simulink model "three_phase_npc_inverter"  (R2021a)
settings: Solver=ode4  StartTime=0.0  StopTime=0.1  FixedStep=1e-6  RelTol=1e-3
libraries: spsIGBTDiodeLib x12, spsDiodeLib x6, simulink x6, spsGroundLib x3, spsDCVoltageSourceLib x2, spsNeutralLib x1, spsThreePhaseSeriesRLCBranchLib x1, spsThreePhaseVIMeasurementLib x1, spspowerguiLib x1
settings Model: Creator=PRANAY KAMAL  LastModifiedBy=PRANAY KAMAL
settings DataIOCC: ReturnWorkspaceOutputs=off

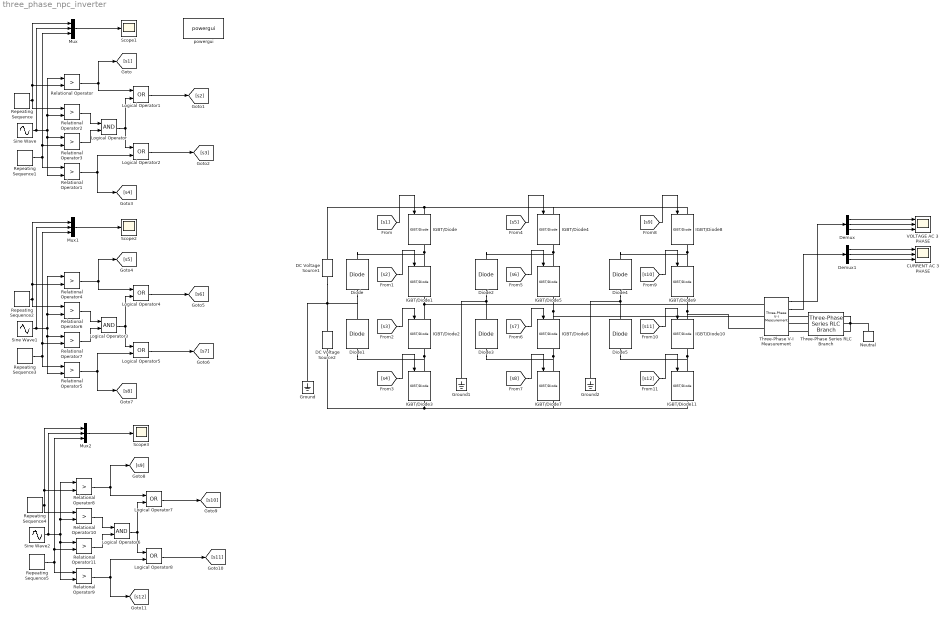
== system three_phase_npc_inverter ==
  CURRENT AC 3 PHASE : Scope  NumInputPorts=3
  DC Voltage Source1 : spsDCVoltageSourceLib/DC Voltage Source  Amplitude=200  Measurements=None
  DC Voltage Source2 : spsDCVoltageSourceLib/DC Voltage Source  Amplitude=200  Measurements=None
  Demux : Demux  Outputs=3
  Demux1 : Demux  Outputs=3
  Diode{,1..5} (6 alike) : spsDiodeLib/Diode  Ron=0.001  Lon=0  Vf=0.8  IC=0  UseSnubber=0  Rs=500  Cs=250e-9  Measurements=off
  Ground : spsGroundLib/Ground  LConnTagsString=a
  Ground1 : spsGroundLib/Ground  LConnTagsString=a
  Ground2 : spsGroundLib/Ground  LConnTagsString=a
  IGBT/Diode{,1..11} (12 alike) : spsIGBTDiodeLib/IGBT//Diode  Ron=1e-3  Rs=1e5  Cs=inf  Measurements=on
  Logical Operator : Logic  AllPortsSameDT=off  OutDataTypeStr=boolean
  Logical Operator{1..2,4..5,7..8} (6 alike) : Logic  Operator=OR  AllPortsSameDT=off  OutDataTypeStr=boolean
  Logical Operator3 : Logic  AllPortsSameDT=off  OutDataTypeStr=boolean
  Logical Operator6 : Logic  AllPortsSameDT=off  OutDataTypeStr=boolean
  Mux : Mux  Inputs=3
  Mux1 : Mux  Inputs=3
  Mux2 : Mux  Inputs=3
  Neutral : spsNeutralLib/Neutral  LConnTagsString=a  NodeNumber=10
      settings: AttributesFormatString=node %<NodeNumber>  SourceProductBaseCode=PS
  Relational Operator{,1..11} (12 alike) : RelationalOperator  Operator=>  OutDataTypeStr=boolean  RndMeth=Simplest
  Repeating Sequence : simulink/Sources/Repeating Sequence  rep_seq_t=[0 0.5 1]*(1/6000)  rep_seq_y=[1 0 1]
  Repeating Sequence1 : simulink/Sources/Repeating Sequence  rep_seq_t=[0 0.5 1]*(1/6000)  rep_seq_y=[0 -1 0]
  Repeating Sequence2 : simulink/Sources/Repeating Sequence  rep_seq_t=[0 0.5 1]*(1/6000)  rep_seq_y=[1 0 1]
  Repeating Sequence3 : simulink/Sources/Repeating Sequence  rep_seq_t=[0 0.5 1]*(1/6000)  rep_seq_y=[0 -1 0]
  Repeating Sequence4 : simulink/Sources/Repeating Sequence  rep_seq_t=[0 0.5 1]*(1/6000)  rep_seq_y=[1 0 1]
  Repeating Sequence5 : simulink/Sources/Repeating Sequence  rep_seq_t=[0 0.5 1]*(1/6000)  rep_seq_y=[0 -1 0]
  Scope1 : Scope
  Scope2 : Scope
  Scope3 : Scope
  Sine Wave : Sin  Amplitude=0.8  Frequency=2*pi*60  SampleTime=0
  Sine Wave1 : Sin  Amplitude=0.8  Frequency=2*pi*60  Phase=2*pi/3  SampleTime=0
  Sine Wave2 : Sin  Amplitude=0.8  Frequency=2*pi*60  Phase=-2*pi/3  SampleTime=0
  Three-Phase Series RLC Branch : spsThreePhaseSeriesRLCBranchLib/Three-Phase Series RLC Branch  LConnTagsString=A|B|C  RConnTagsString=A|B|C  BranchType=RL  Resistance=0.1  Inductance=1e-2  Capacitance=1e-6  Measurements=None
  Three-Phase V-I Measurement : spsThreePhaseVIMeasurementLib/Three-Phase V-I Measurement  VoltageMeasurement=phase-to-ground  SetLabelV=off  LabelV=Vabc  Vpu=off  VpuLL=off  CurrentMeasurement=yes  SetLabelI=off  LabelI=Iabc  Ipu=off  Pbase=100e6  Vbase=500e3  OutputType=Complex  PhasorSimulation=off  PSBequivalent=0
  VOLTAGE AC 3 PHASE : Scope  NumInputPorts=3
  powergui : spspowerguiLib/powergui  Priority=1  SimulationMode=Discrete  SampleTime=1e-6  frequency=60  Iterations=50  frequencyindice=0  Pbase=100e6  ErrMax=1e-4  UnitsV=kV  UnitsW=MW  buscounter=0  FunctionMessages=off  echomessages=off  EnableUseOfTLC=off  CurrentSourceSwitches=off  DisableSnubberDevices=off  DisableRonSwitches=off  DisableVfSwitches=off  DisplayEquations=off  AutomaticDiscreteSolvers=off  SolverType=Tustin/Backward Euler (TBE)  Interpol=off  ExternalGateDelay=off  methode=off  Ts=100  x0status=blocks  SPID=on  SwTol=0  HookPort=off  NonlinearTolerance=1e-4  nMaxIteration=100  ContinueOnMaxIteration=off  RestoreLinks=warning  ResistiveCurrentMeasurement=off  Frange=[0:2:500]  Ylog=off  Xlog=on  ShowGrid=off  save=off  variable=ZData  structure=0  ZoomFFT=off  StartTime=0.0  cycles=1  DisplayStyle=1  fundamental=60  FreqAxis=off  MaxFrequency=1000  frequencyindicesteady=1  RmsSteady=1  display=off
  wires:
  Relational Operator3/1 -> Logical Operator/2
  Relational Operator/1 -> Logical Operator1/1, [s1]
  [s1] -> IGBT/Diode/1
  Repeating Sequence/1 -> Relational Operator2/1, Mux/1, Relational Operator/2
  [s3] -> IGBT/Diode2/1
  [s2] -> IGBT/Diode1/1
  Repeating Sequence1/1 -> Relational Operator1/1, Relational Operator3/2, Mux/3
  Sine Wave/1 -> Mux/2, Relational Operator1/2, Relational Operator3/1, Relational Operator2/2, Relational Operator/1
  [s4] -> IGBT/Diode3/1
  Relational Operator2/1 -> Logical Operator/1
  Logical Operator1/1 -> [s2]
  Logical Operator/1 -> Logical Operator2/1, Logical Operator1/2
  Logical Operator2/1 -> [s3]
  Relational Operator1/1 -> [s4], Logical Operator2/2
  Mux/1 -> Scope1/1
  [s5] -> IGBT/Diode4/1
  [s6] -> IGBT/Diode5/1
  [s8] -> IGBT/Diode7/1
  [s7] -> IGBT/Diode6/1
  [s12] -> IGBT/Diode11/1
  [s9] -> IGBT/Diode8/1
  [s11] -> IGBT/Diode10/1
  [s10] -> IGBT/Diode9/1
  Logical Operator3/1 -> Logical Operator5/1, Logical Operator4/2
  Logical Operator5/1 -> [s7]
  Logical Operator4/1 -> [s6]
  Sine Wave1/1 -> Mux1/2, Relational Operator5/2, Relational Operator7/1, Relational Operator6/2, Relational Operator4/1
  Mux1/1 -> Scope2/1
  Relational Operator6/1 -> Logical Operator3/1
  Repeating Sequence3/1 -> Relational Operator5/1, Relational Operator7/2, Mux1/3
  Relational Operator5/1 -> [s8], Logical Operator5/2
  Relational Operator4/1 -> Logical Operator4/1, [s5]
  Relational Operator7/1 -> Logical Operator3/2
  Repeating Sequence2/1 -> Relational Operator6/1, Mux1/1, Relational Operator4/2
  Logical Operator6/1 -> Logical Operator8/1, Logical Operator7/2
  Logical Operator8/1 -> [s11]
  Logical Operator7/1 -> [s10]
  Sine Wave2/1 -> Mux2/2, Relational Operator9/2, Relational Operator11/1, Relational Operator10/2, Relational Operator8/1
  Mux2/1 -> Scope3/1
  Relational Operator10/1 -> Logical Operator6/1
  Repeating Sequence5/1 -> Relational Operator9/1, Relational Operator11/2, Mux2/3
  Relational Operator9/1 -> [s12], Logical Operator8/2
  Relational Operator8/1 -> Logical Operator7/1, [s9]
  Relational Operator11/1 -> Logical Operator6/2
  Repeating Sequence4/1 -> Relational Operator10/1, Mux2/1, Relational Operator8/2
  Demux1/2 -> CURRENT AC 3 PHASE/2
  Demux1/1 -> CURRENT AC 3 PHASE/1
  Demux/3 -> VOLTAGE AC 3 PHASE/3
  Demux/1 -> VOLTAGE AC 3 PHASE/1
  Demux/2 -> VOLTAGE AC 3 PHASE/2
  Demux1/3 -> CURRENT AC 3 PHASE/3
  Three-Phase V-I Measurement/1 -> Demux/1
  Three-Phase V-I Measurement/2 -> Demux1/1
  connections:
  IGBT/Diode2/RConn1 -- IGBT/Diode3/LConn1 -- Diode1/LConn1
  Ground/LConn1 -- DC Voltage Source2/RConn1 -- DC Voltage Source1/LConn1 -- Diode1/RConn1 -- Diode/LConn1
  IGBT/Diode/RConn1 -- IGBT/Diode1/LConn1 -- Diode/RConn1
  IGBT/Diode2/LConn1 -- Three-Phase V-I Measurement/LConn1 -- IGBT/Diode1/RConn1
  DC Voltage Source1/RConn1 -- IGBT/Diode8/LConn1 -- IGBT/Diode4/LConn1 -- IGBT/Diode/LConn1
  DC Voltage Source2/LConn1 -- IGBT/Diode11/RConn1 -- IGBT/Diode7/RConn1 -- IGBT/Diode3/RConn1
  Diode2/LConn1 -- Ground1/LConn1 -- Diode3/RConn1
  IGBT/Diode4/RConn1 -- IGBT/Diode5/LConn1 -- Diode2/RConn1
  IGBT/Diode6/RConn1 -- IGBT/Diode7/LConn1 -- Diode3/LConn1
  IGBT/Diode6/LConn1 -- IGBT/Diode5/RConn1 -- Three-Phase V-I Measurement/LConn2
  IGBT/Diode8/RConn1 -- IGBT/Diode9/LConn1 -- Diode4/RConn1
  Diode4/LConn1 -- Ground2/LConn1 -- Diode5/RConn1
  IGBT/Diode10/RConn1 -- IGBT/Diode11/LConn1 -- Diode5/LConn1
  IGBT/Diode10/LConn1 -- IGBT/Diode9/RConn1 -- Three-Phase V-I Measurement/LConn3
  Three-Phase Series RLC Branch/LConn1 -- Three-Phase V-I Measurement/RConn1
  Three-Phase Series RLC Branch/LConn2 -- Three-Phase V-I Measurement/RConn2
  Three-Phase Series RLC Branch/LConn3 -- Three-Phase V-I Measurement/RConn3
  Three-Phase Series RLC Branch/RConn1 -- Neutral/LConn1 -- Three-Phase Series RLC Branch/RConn2 -- Three-Phase Series RLC Branch/RConn3
